simulink subsystem "model_6dof"  (R2025b)
settings: Solver=VariableStepAuto  StartTime=0.0  StopTime=10.0  RelTol=1e-3
values from neighbouring files (symbols this model uses):
  a = 13.06    [params.m]    (also in params_3dof.m = 13; test.m = 0.0013)
  b = 0.0859    [params.m]    (also in params_3dof.m = 0.085908; test.m = 8.5908)
  E = [ ... (first row only)    [params_3dof.m]    (also in test.m)
  g = 9.81    [params.m]    (also in params_1dof.m; params_3dof.m)
  I = diag([I_xx, I_yy, I_zz])    [params_3dof.m]
  m = 1.210    (= 1.21)    [params.m]    (also in params_1dof.m = 1.014; params_3dof.m = 1.114)
  p = [p_x, p_y, p_z]    [params.m]    (also in params_3dof.m = 0.05)
  T_delay_actor = 0    [params.m]    (also in params_3dof.m)
settings Model: Creator=schwmaxi  LastModifiedBy=schwmaxi

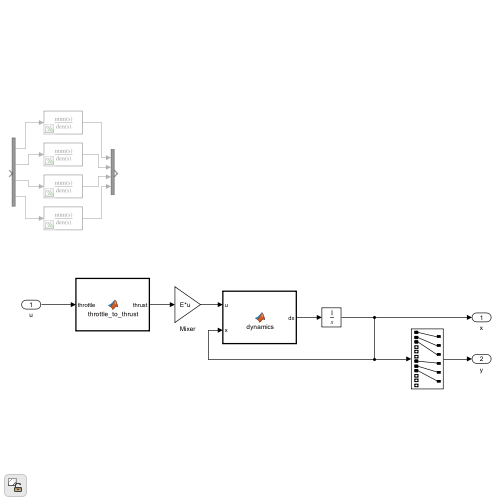
[thumbnail: Simulink's stored preview of the top-level diagram]
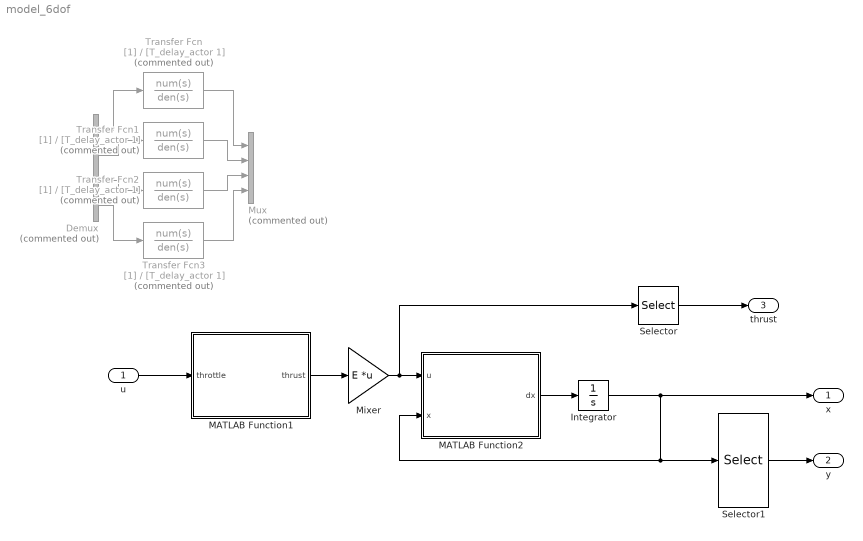
== system model_6dof ==
  u : Inport  OutDataTypeStr=double  PortDimensions=4  SampleTime=0
  Demux : Demux  Commented=on
  Integrator : Integrator  InitialCondition=[0; 0; 0; 0; 0; 0; 0; 0; 0; 0; 0; 0]
  MATLAB Function1 : MATLAB Function  TreatAsAtomicUnit=on
  MATLAB Function2 : MATLAB Function  TreatAsAtomicUnit=on
  Mixer : Gain  Gain=E  Multiplication=Matrix(K*u)
  Mux : Mux  Commented=on
  Selector : Selector  InputPortWidth=4  IndexOptions=Index vector (dialog)  Indices=[1]  OutputSizes=1
  Selector1 : Selector  InputPortWidth=12  IndexOptions=Index vector (dialog)  Indices=[1 2 3 7 8 9]  OutputSizes=1
  Transfer Fcn{,1..3} (4 alike) : TransferFcn  Commented=on  Denominator=[T_delay_actor 1]
  x : Outport  OutDataTypeStr=double  SampleTime=0
  y : Outport  Port=2  OutDataTypeStr=double  SampleTime=0
  thrust : Outport  Port=3
  wires:
  Mixer/1 -> MATLAB Function2/1(u), Selector/1
  MATLAB Function2/1(dx) -> Integrator/1
  MATLAB Function1/1(thrust) -> Mixer/1
  Transfer Fcn/1 -> Mux/1
  Demux/4 -> Transfer Fcn3/1
  Demux/1 -> Transfer Fcn/1
  Transfer Fcn3/1 -> Mux/4
  Transfer Fcn2/1 -> Mux/3
  Demux/3 -> Transfer Fcn2/1
  Transfer Fcn1/1 -> Mux/2
  Demux/2 -> Transfer Fcn1/1
  u/1 -> MATLAB Function1/1(throttle)
  Integrator/1 -> x/1, MATLAB Function2/2(x), Selector1/1
  Selector1/1 -> y/1
  Selector/1 -> thrust/1

== matlab function model_6dof/MATLAB Function1 ==
  data: thrust output; throttle input; a parameter; b parameter
function thrust = throttle_to_thrust(throttle, a, b)
    thrust = a * (throttle - b).^2;
end

== matlab function model_6dof/MATLAB Function2 ==
  data: u input; x input; dx output; I parameter; p parameter; m parameter; g parameter
function dx = dynamics(u, x, I, p, m, g)
    % I und p wird als Parameter Data übergeben, vgl. Symbols Pane
    thrust = u(1);
    torques = u(2:4);

    phi = x(7);
    theta = x(8);
    psi = x(9);

    omega = x(10:12);

    % Elementarmatrizen
    R_x = [1, 0, 0; 
           0, cos(phi), -sin(phi); 
           0, sin(phi), cos(phi)];
    
    R_y = [cos(theta), 0, sin(theta); 
           0, 1, 0; 
           -sin(theta), 0, cos(theta)];
    
    R_z = [cos(psi), -sin(psi), 0; 
           sin(psi), cos(psi), 0; 
           0, 0, 1];

    % Gesamt-Rotationsmatrix (Body to World: R = Rz * Ry * Rx)
    R = R_z * R_y * R_x;

    position_dot = x(4:6);
    velocity_dot = [0; 0; g] +1/m * R * [0; 0; -thrust];

    body_to_euler_rates = [
        1, sin(phi) * tan(theta), cos(phi)*tan(theta);
        0, cos(phi), -sin(phi);
        0, sin(phi) / cos(theta), cos(phi)/cos(theta);
    ];
    
    damping_moments = p * omega;

    angles_dot = body_to_euler_rates * omega(:);
    omega_dot = I \ (torques - damping_moments - cross(omega, I * omega));

    dx = [position_dot; velocity_dot; angles_dot; omega_dot];
end
